simulink model "PassengerCar"  (R2019b)
settings: Solver=ode1  StartTime=0  StopTime=25  FixedStep=1.0000000000000000e-003  RelTol=1e-3
InitFcn:
  | sampleTime = str2double(get_param(bdroot, 'FixedStep'));
undefined symbols (not defined in the file or in its folder): AccPedalPos, BrakePedalPos, BrakeSwitch, DiscIntNeverNeededParam, DYNA4, EngSpd, IgnitionSwitch, InitialGear, InitialSpeed, IntendedEngTrq, LeftIndicator, MainBrakePress, MaxGear, MDL, MinGear, RefAcc, RefLane, RefLatPos, RefPath, RefPathCurv, RefSpd, RefSpdPreview, RefSpdRetrospect, RightIndicator, SteeringWheelAng, SteeringWheelTrq, UserDefinedRefValue, vm_const
libraries: UtilitiesLibrary x31, simulink x18, WheelSystemModules x13, LongitudinalControllerModules x13, LateralControllerModules x7, AnimationBusselectorModules x5, EnvironmentModules x5, BasicEngineControlModules x5, MiscellaneousControlModules x5, Animation3Modules x4, AuxiliariesModules x4, TireModules x4
(part 19 of 39)

== system PassengerCar/Vehicle/Engine/EngineControlUnit/EngineControlUnitOutput ==
  StarterSwitch[0;1]___UNIQUE_1 : Inport  Description=|  PortDimensions=[1]
      | <name>StarterSwitch[0;1]</name>
      | <comment>Engine starter switch</comment>
  EngRunPermission[0;1]___UNIQUE_1 : Inport  Description=|  Port=2  PortDimensions=[1]
      | <name>EngRunPermission[0;1]</name>
      | <comment>Switch indicating a engine stop due to start stop function or ignition off</comment>
  EngLoadSignal[0_1]___UNIQUE_1 : Inport  Description=|  Port=3  PortDimensions=[1]
      | <name>EngLoadSignal[0_1]</name>
      | <comment>Engine load signal</comment>
  EngIdleSpd[rad/s]___UNIQUE_1 : Inport  Description=|  Port=4  PortDimensions=[1]
      | <name>EngIdleSpd[rad/s]</name>
      | <comment>Engine idle speed</comment>
  EngFuelCutoff[0;1]___UNIQUE_1 : Inport  Description=|  Port=5  PortDimensions=[1]
      | <name>EngFuelCutoff[0;1]</name>
      | <comment>Logical signal which is true if fuel mass flow is stopped</comment>
  MaxEngSpd[rad/s]___UNIQUE_1 : Inport  Description=|  Port=6  PortDimensions=[1]
      | <name>MaxEngSpd[rad/s]</name>
      | <comment>Maximum allowed engine speed, threshold for fuel cut off</comment>
  UpperEngTrqSwitch[0;2]___UNIQUE_1 : Inport  Description=|  Port=7  PortDimensions=[1]
      | <name>UpperEngTrqSwitch[0;2]</name>
      | <comment>Switch indicating how the upper engine torque should be restricted (0: off, 1: slow, 2: fast)</comment>
  UpperEngTrqLimit[Nm]___UNIQUE_1 : Inport  Description=|  Port=8  PortDimensions=[1]
      | <name>UpperEngTrqLimit[Nm]</name>
      | <comment>Upper limit for the engine torque</comment>
  LowerEngTrqSwitch[0;2]___UNIQUE_1 : Inport  Description=|  Port=9  PortDimensions=[1]
      | <name>LowerEngTrqSwitch[0;2]</name>
      | <comment>Switch indicating how the lower engine torque should be restricted (0: off, 1: slow, 2: fast)</comment>
  LowerEngTrqLimit[Nm]___UNIQUE_1 : Inport  Description=|  Port=10  PortDimensions=[1]
      | <name>LowerEngTrqLimit[Nm]</name>
      | <comment>Lower limit for the engine torque</comment>
  __TDD__EngineControlUnit.EngFuelCutoff[0;1] : Demux  Outputs=[1]
  __TDD__EngineControlUnit.EngIdleSpd[rad/s] : Demux  Outputs=[1]
  __TDD__EngineControlUnit.EngLoadSignal[0_1] : Demux  Outputs=[1]
  __TDD__EngineControlUnit.EngRunPermission[0;1] : Demux  Outputs=[1]
  __TDD__EngineControlUnit.LowerEngTrqLimit[Nm] : Demux  Outputs=[1]
  __TDD__EngineControlUnit.LowerEngTrqSwitch[0;2] : Demux  Outputs=[1]
  __TDD__EngineControlUnit.MaxEngSpd[rad/s] : Demux  Outputs=[1]
  __TDD__EngineControlUnit.StarterSwitch[0;1] : Demux  Outputs=[1]
  __TDD__EngineControlUnit.UpperEngTrqLimit[Nm] : Demux  Outputs=[1]
  __TDD__EngineControlUnit.UpperEngTrqSwitch[0;2] : Demux  Outputs=[1]
  __TDO__EngineControlUnit : BusCreator  Inputs=10
  EngineControlUnit___UNIQUE_1 : Outport  Description=|  PortDimensions=[10]  VectorParamsAs1DForOutWhenUnconnected=off
      | <name>StarterSwitch[0;1]</name>
      | <comment>Engine starter switch</comment>
  wires:
  __TDO__EngineControlUnit/1 -> EngineControlUnit___UNIQUE_1/1  "EngineControlUnit"
  __TDD__EngineControlUnit.LowerEngTrqLimit[Nm]/1 -> __TDO__EngineControlUnit/10  "LowerEngTrqLimit[Nm]"
  LowerEngTrqLimit[Nm]___UNIQUE_1/1 -> __TDD__EngineControlUnit.LowerEngTrqLimit[Nm]/1
  __TDD__EngineControlUnit.LowerEngTrqSwitch[0;2]/1 -> __TDO__EngineControlUnit/9  "LowerEngTrqSwitch[0;2]"
  LowerEngTrqSwitch[0;2]___UNIQUE_1/1 -> __TDD__EngineControlUnit.LowerEngTrqSwitch[0;2]/1
  __TDD__EngineControlUnit.UpperEngTrqLimit[Nm]/1 -> __TDO__EngineControlUnit/8  "UpperEngTrqLimit[Nm]"
  UpperEngTrqLimit[Nm]___UNIQUE_1/1 -> __TDD__EngineControlUnit.UpperEngTrqLimit[Nm]/1
  __TDD__EngineControlUnit.UpperEngTrqSwitch[0;2]/1 -> __TDO__EngineControlUnit/7  "UpperEngTrqSwitch[0;2]"
  UpperEngTrqSwitch[0;2]___UNIQUE_1/1 -> __TDD__EngineControlUnit.UpperEngTrqSwitch[0;2]/1
  __TDD__EngineControlUnit.MaxEngSpd[rad/s]/1 -> __TDO__EngineControlUnit/6  "MaxEngSpd[rad/s]"
  MaxEngSpd[rad/s]___UNIQUE_1/1 -> __TDD__EngineControlUnit.MaxEngSpd[rad/s]/1
  __TDD__EngineControlUnit.EngFuelCutoff[0;1]/1 -> __TDO__EngineControlUnit/5  "EngFuelCutoff[0;1]"
  EngFuelCutoff[0;1]___UNIQUE_1/1 -> __TDD__EngineControlUnit.EngFuelCutoff[0;1]/1
  __TDD__EngineControlUnit.EngIdleSpd[rad/s]/1 -> __TDO__EngineControlUnit/4  "EngIdleSpd[rad/s]"
  EngIdleSpd[rad/s]___UNIQUE_1/1 -> __TDD__EngineControlUnit.EngIdleSpd[rad/s]/1
  __TDD__EngineControlUnit.EngLoadSignal[0_1]/1 -> __TDO__EngineControlUnit/3  "EngLoadSignal[0_1]"
  EngLoadSignal[0_1]___UNIQUE_1/1 -> __TDD__EngineControlUnit.EngLoadSignal[0_1]/1
  __TDD__EngineControlUnit.EngRunPermission[0;1]/1 -> __TDO__EngineControlUnit/2  "EngRunPermission[0;1]"
  EngRunPermission[0;1]___UNIQUE_1/1 -> __TDD__EngineControlUnit.EngRunPermission[0;1]/1
  __TDD__EngineControlUnit.StarterSwitch[0;1]/1 -> __TDO__EngineControlUnit/1  "StarterSwitch[0;1]"
  StarterSwitch[0;1]___UNIQUE_1/1 -> __TDD__EngineControlUnit.StarterSwitch[0;1]/1

== system PassengerCar/Vehicle/Engine/EngineControlUnit/InputFromCTRL ==
  fromCTRL : Inport
  TDBusSelector : BusSelector  OutputSignals=CTRL.LongitudinalControl.IgnitionSwitch[0;3],CTRL.LongitudinalControl.EngRunPermission[0;1],CTRL.LongitudinalControl.AccPedalPos[0_1],CTRL.LongitudinalControl.IntendedEngTrq[Nm],CTRL.LongitudinalControl.IntendedEngTrqActive[0;1],CTRL.LongitudinalControl.ClutchPos[0_1]
  __TDD__AccPedalPos[0_1] : Demux  Outputs=1
  __TDD__ClutchPos[0_1] : Demux  Outputs=[1]
  __TDD__EngRunPermission[0;1] : Demux  Outputs=[1]
  __TDD__IgnitionSwitch[0;3] : Demux  Outputs=[1]
  __TDD__IntendedEngTrqActive[0;1] : Demux  Outputs=[1]
  __TDD__IntendedEngTrq[Nm] : Demux  Outputs=[1]
  IgnitionSwitch[0;3]___UNIQUE_1 : Outport  Description=|  PortDimensions=[1]  VectorParamsAs1DForOutWhenUnconnected=off
      | <name>CTRL.LongitudinalControl.IgnitionSwitch[0;3]</name>
      | <comment>Ignition signal with four signal states: 0 - ignition off + consumer off + starter off, 1 - ignition off + consumer on + starter off, 2 - ignition on + consumer on + starter off, 3 - ignition on + consumer on  + starter on</comment>
  EngRunPermission[0;1]___UNIQUE_1 : Outport  Description=|  Port=2  PortDimensions=[1]  VectorParamsAs1DForOutWhenUnconnected=off
      | <name>CTRL.LongitudinalControl.EngRunPermission[0;1]</name>
      | <comment></comment>
  AccPedalPos[0_1]___UNIQUE_1 : Outport  Description=|  Port=3  VectorParamsAs1DForOutWhenUnconnected=off
      | <name>CTRL.LongitudinalControl.AccPedalPos[0_1]</name>
      | <comment></comment>
  IntendedEngTrq[Nm]___UNIQUE_1 : Outport  Description=|  Port=4  PortDimensions=[1]  VectorParamsAs1DForOutWhenUnconnected=off
      | <name>CTRL.LongitudinalControl.IntendedEngTrq[Nm]</name>
      | <comment></comment>
  IntendedEngTrqActive[0;1]___UNIQUE_1 : Outport  Description=|  Port=5  PortDimensions=[1]  VectorParamsAs1DForOutWhenUnconnected=off
      | <name>CTRL.LongitudinalControl.IntendedEngTrqActive[0;1]</name>
      | <comment></comment>
  ClutchPos[0_1]___UNIQUE_1 : Outport  Description=|  Port=6  PortDimensions=[1]  VectorParamsAs1DForOutWhenUnconnected=off
      | <name>CTRL.LongitudinalControl.ClutchPos[0_1]</name>
      | <comment>Clutch position</comment>
  wires:
  __TDD__ClutchPos[0_1]/1 -> ClutchPos[0_1]___UNIQUE_1/1  "ClutchPos[0_1]"
  __TDD__IntendedEngTrqActive[0;1]/1 -> IntendedEngTrqActive[0;1]___UNIQUE_1/1  "IntendedEngTrqActive[0;1]"
  __TDD__IntendedEngTrq[Nm]/1 -> IntendedEngTrq[Nm]___UNIQUE_1/1  "IntendedEngTrq[Nm]"
  __TDD__AccPedalPos[0_1]/1 -> AccPedalPos[0_1]___UNIQUE_1/1  "AccPedalPos[0_1]"
  __TDD__EngRunPermission[0;1]/1 -> EngRunPermission[0;1]___UNIQUE_1/1  "EngRunPermission[0;1]"
  __TDD__IgnitionSwitch[0;3]/1 -> IgnitionSwitch[0;3]___UNIQUE_1/1  "IgnitionSwitch[0;3]"
  TDBusSelector/6 -> __TDD__ClutchPos[0_1]/1  "<ClutchPos[0_1]>"
  TDBusSelector/5 -> __TDD__IntendedEngTrqActive[0;1]/1  "<IntendedEngTrqActive[0;1]>"
  TDBusSelector/4 -> __TDD__IntendedEngTrq[Nm]/1  "<IntendedEngTrq[Nm]>"
  TDBusSelector/3 -> __TDD__AccPedalPos[0_1]/1  "<AccPedalPos[0_1]>"
  TDBusSelector/2 -> __TDD__EngRunPermission[0;1]/1  "<EngRunPermission[0;1]>"
  TDBusSelector/1 -> __TDD__IgnitionSwitch[0;3]/1  "<IgnitionSwitch[0;3]>"
  fromCTRL/1 -> TDBusSelector/1

== system PassengerCar/Vehicle/Engine/EngineControlUnit/InputFromCTRL1 ==
  fromCTRL : Inport
  TDBusSelector : BusSelector  OutputSignals=CTRL.LongitudinalControl.ASRRequestSwitch[0;2],CTRL.LongitudinalControl.ASRTrq[Nm],CTRL.LongitudinalControl.MSRRequestSwitch[0;2],CTRL.LongitudinalControl.MSRTrq[Nm]
  __TDD__ASRRequestSwitch[0;2] : Demux  Outputs=1
  __TDD__ASRTrq[Nm] : Demux  Outputs=1
  __TDD__MSRRequestSwitch[0;2] : Demux  Outputs=1
  __TDD__MSRTrq[Nm] : Demux  Outputs=1
  ASRRequestSwitch[0;2]___UNIQUE_1 : Outport  Description=|  VectorParamsAs1DForOutWhenUnconnected=off
      | <name>CTRL.LongitudinalControl.ASRRequestSwitch[0;2]</name>
      | <comment></comment>
  ASRTrq[Nm]___UNIQUE_1 : Outport  Description=|  Port=2  VectorParamsAs1DForOutWhenUnconnected=off
      | <name>CTRL.LongitudinalControl.ASRTrq[Nm]</name>
      | <comment></comment>
  MSRRequestSwitch[0;2]___UNIQUE_1 : Outport  Description=|  Port=3  VectorParamsAs1DForOutWhenUnconnected=off
      | <name>CTRL.LongitudinalControl.MSRRequestSwitch[0;2]</name>
      | <comment></comment>
  MSRTrq[Nm]___UNIQUE_1 : Outport  Description=|  Port=4  VectorParamsAs1DForOutWhenUnconnected=off
      | <name>CTRL.LongitudinalControl.MSRTrq[Nm]</name>
      | <comment></comment>
  wires:
  __TDD__MSRTrq[Nm]/1 -> MSRTrq[Nm]___UNIQUE_1/1  "MSRTrq[Nm]"
  __TDD__MSRRequestSwitch[0;2]/1 -> MSRRequestSwitch[0;2]___UNIQUE_1/1  "MSRRequestSwitch[0;2]"
  __TDD__ASRTrq[Nm]/1 -> ASRTrq[Nm]___UNIQUE_1/1  "ASRTrq[Nm]"
  __TDD__ASRRequestSwitch[0;2]/1 -> ASRRequestSwitch[0;2]___UNIQUE_1/1  "ASRRequestSwitch[0;2]"
  TDBusSelector/4 -> __TDD__MSRTrq[Nm]/1  "<MSRTrq[Nm]>"
  TDBusSelector/3 -> __TDD__MSRRequestSwitch[0;2]/1  "<MSRRequestSwitch[0;2]>"
  TDBusSelector/2 -> __TDD__ASRTrq[Nm]/1  "<ASRTrq[Nm]>"
  TDBusSelector/1 -> __TDD__ASRRequestSwitch[0;2]/1  "<ASRRequestSwitch[0;2]>"
  fromCTRL/1 -> TDBusSelector/1

== system PassengerCar/Vehicle/Engine/EngineControlUnit/InputFromChassis ==
  fromChassis : Inport
  TDBusSelector : BusSelector  OutputSignals=VehicleBody.AbsVel[m/s]
  __TDD__AbsVel[m/s] : Demux  Outputs=1
  AbsVel[m/s]___UNIQUE_1 : Outport  Description=|  VectorParamsAs1DForOutWhenUnconnected=off
      | <name>VehicleBody.AbsVel[m/s]</name>
      | <comment></comment>
  wires:
  __TDD__AbsVel[m/s]/1 -> AbsVel[m/s]___UNIQUE_1/1  "AbsVel[m/s]"
  TDBusSelector/1 -> __TDD__AbsVel[m/s]/1  "<AbsVel[m/s]>"
  fromChassis/1 -> TDBusSelector/1

== system PassengerCar/Vehicle/Engine/EngineControlUnit/InputFromDrivetrain ==
  fromDrivetrain : Inport
  TDBusSelector : BusSelector  OutputSignals=DrivetrainPhysics.Transmission.Gear[-4;20],DrivetrainPhysics.EngSpd[rad/s]
  __TDD__EngSpd[rad/s] : Demux  Outputs=1
  __TDD__Gear[-4;20] : Demux  Outputs=1
  Gear[-4;20] : Outport  Description=|  VectorParamsAs1DForOutWhenUnconnected=off
      | <name>DrivetrainPhysics.Transmission.Gear[-4;20]</name>
      | <comment></comment>
  EngSpd[rad/s] : Outport  Description=|  Port=2  VectorParamsAs1DForOutWhenUnconnected=off
      | <name>DrivetrainPhysics.EngSpd[rad/s]</name>
      | <comment></comment>
  wires:
  __TDD__EngSpd[rad/s]/1 -> EngSpd[rad/s]/1  "EngSpd[rad/s]"
  __TDD__Gear[-4;20]/1 -> Gear[-4;20]/1  "Gear[-4;20]"
  TDBusSelector/2 -> __TDD__EngSpd[rad/s]/1  "<EngSpd[rad/s]>"
  TDBusSelector/1 -> __TDD__Gear[-4;20]/1  "<Gear[-4;20]>"
  fromDrivetrain/1 -> TDBusSelector/1

== system PassengerCar/Vehicle/Engine/EngineControlUnit/InputFromEnginePhysics ==
  fromEnginePhysics : Inport
  TDBusSelector : BusSelector  OutputSignals=Mechanics.EngTrq[Nm],Mechanics.UnrestrictedEngTrq[Nm],Mechanics.MeanEngFrictionTrq[Nm],Mechanics.MeanEngMaxTrq[Nm]
  __TDD__EngTrq[Nm] : Demux  Outputs=[1]
  __TDD__MeanEngFrictionTrq[Nm] : Demux  Outputs=1
  __TDD__MeanEngMaxTrq[Nm] : Demux  Outputs=1
  __TDD__UnrestrictedEngTrq[Nm] : Demux  Outputs=[1]
  EngTrq[Nm]___UNIQUE_1 : Outport  Description=|  PortDimensions=[1]  VectorParamsAs1DForOutWhenUnconnected=off
      | <name>Mechanics.EngTrq[Nm]</name>
      | <comment>Engine torque</comment>
  UnrestrictedEngTrq[Nm]___UNIQUE_1 : Outport  Description=|  Port=2  PortDimensions=[1]  VectorParamsAs1DForOutWhenUnconnected=off
      | <name>Mechanics.UnrestrictedEngTrq[Nm]</name>
      | <comment>Unrestricted engine torque</comment>
  MeanEngFrictionTrq[Nm]___UNIQUE_1 : Outport  Description=|  Port=3  VectorParamsAs1DForOutWhenUnconnected=off
      | <name>Mechanics.MeanEngFrictionTrq[Nm]</name>
      | <comment></comment>
  MeanEngMaxTrq[Nm]___UNIQUE_1 : Outport  Description=|  Port=4  VectorParamsAs1DForOutWhenUnconnected=off
      | <name>Mechanics.MeanEngMaxTrq[Nm]</name>
      | <comment></comment>
  wires:
  __TDD__MeanEngMaxTrq[Nm]/1 -> MeanEngMaxTrq[Nm]___UNIQUE_1/1  "MeanEngMaxTrq[Nm]"
  __TDD__MeanEngFrictionTrq[Nm]/1 -> MeanEngFrictionTrq[Nm]___UNIQUE_1/1  "MeanEngFrictionTrq[Nm]"
  __TDD__UnrestrictedEngTrq[Nm]/1 -> UnrestrictedEngTrq[Nm]___UNIQUE_1/1  "UnrestrictedEngTrq[Nm]"
  __TDD__EngTrq[Nm]/1 -> EngTrq[Nm]___UNIQUE_1/1  "EngTrq[Nm]"
  TDBusSelector/4 -> __TDD__MeanEngMaxTrq[Nm]/1  "<MeanEngMaxTrq[Nm]>"
  TDBusSelector/3 -> __TDD__MeanEngFrictionTrq[Nm]/1  "<MeanEngFrictionTrq[Nm]>"
  TDBusSelector/2 -> __TDD__UnrestrictedEngTrq[Nm]/1  "<UnrestrictedEngTrq[Nm]>"
  TDBusSelector/1 -> __TDD__EngTrq[Nm]/1  "<EngTrq[Nm]>"
  fromEnginePhysics/1 -> TDBusSelector/1

== system PassengerCar/Vehicle/Engine/EnginePhysics/DynaComponentInfo ==

== system PassengerCar/Vehicle/Engine/EnginePhysics/EnginePhysicsOutput ==
  Mechanics___UNIQUE_1 : Inport  Description=|
      | <name>Mechanics</name>
      | <comment></comment>
  ValidityStatus___UNIQUE_1 : Inport  Description=|  Port=2
      | <name>ValidityStatus</name>
      | <comment></comment>
  FuelSystem___UNIQUE_1 : Inport  Description=|  Port=3
      | <name>FuelSystem</name>
      | <comment></comment>
  __TDO__EnginePhysics : BusCreator  Inputs=3
  EnginePhysics___UNIQUE_1 : Outport  Description=|  VectorParamsAs1DForOutWhenUnconnected=off
      | <name>Mechanics</name>
      | <comment></comment>
  wires:
  __TDO__EnginePhysics/1 -> EnginePhysics___UNIQUE_1/1  "EnginePhysics"
  FuelSystem___UNIQUE_1/1 -> __TDO__EnginePhysics/3  "FuelSystem"
  ValidityStatus___UNIQUE_1/1 -> __TDO__EnginePhysics/2  "ValidityStatus"
  Mechanics___UNIQUE_1/1 -> __TDO__EnginePhysics/1  "Mechanics"

== system PassengerCar/Vehicle/Engine/EnginePhysics/FuelSystemOutput ==
  FuelMassFlow[kg/s]___UNIQUE_1 : Inport  Description=|  PortDimensions=[1]
      | <name>FuelMassFlow[kg/s]</name>
      | <comment></comment>
  FuelMass[kg]___UNIQUE_1 : Inport  Description=|  Port=2  PortDimensions=[1]
      | <name>FuelMass[kg]</name>
      | <comment></comment>
  CurrFuelConsumEu[l/100km]___UNIQUE_1 : Inport  Description=|  Port=3  PortDimensions=[1]
      | <name>CurrFuelConsumEu[l/100km]</name>
      | <comment></comment>
  CurrFuelConsumUs[mpg]___UNIQUE_1 : Inport  Description=|  Port=4  PortDimensions=[1]
      | <name>CurrFuelConsumUs[mpg]</name>
      | <comment></comment>
  AvgFuelConsumEu[l/100km]___UNIQUE_1 : Inport  Description=|  Port=5  PortDimensions=[1]
      | <name>AvgFuelConsumEu[l/100km]</name>
      | <comment></comment>
  AvgFuelConsumUs[mpg]___UNIQUE_1 : Inport  Description=|  Port=6  PortDimensions=[1]
      | <name>AvgFuelConsumUs[mpg]</name>
      | <comment></comment>
  Efficiency[-]___UNIQUE_1 : Inport  Description=|  Port=7  PortDimensions=[1]
      | <name>Efficiency[-]</name>
      | <comment></comment>
  FuelDensity[kg/m**3]___UNIQUE_1 : Inport  Description=|  Port=8  PortDimensions=[1]
      | <name>FuelDensity[kg/m**3]</name>
      | <comment></comment>
  __TDD__FuelSystem.AvgFuelConsumEu[l/100km] : Demux  Outputs=[1]
  __TDD__FuelSystem.AvgFuelConsumUs[mpg] : Demux  Outputs=[1]
  __TDD__FuelSystem.CurrFuelConsumEu[l/100km] : Demux  Outputs=[1]
  __TDD__FuelSystem.CurrFuelConsumUs[mpg] : Demux  Outputs=[1]
  __TDD__FuelSystem.Efficiency[-] : Demux  Outputs=[1]
  __TDD__FuelSystem.FuelDensity[kg/m**3] : Demux  Outputs=[1]
  __TDD__FuelSystem.FuelMassFlow[kg/s] : Demux  Outputs=[1]
  __TDD__FuelSystem.FuelMass[kg] : Demux  Outputs=[1]
  __TDO__FuelSystem : BusCreator  Inputs=8
  FuelSystem___UNIQUE_1 : Outport  Description=|  PortDimensions=[8]  VectorParamsAs1DForOutWhenUnconnected=off
      | <name>FuelMassFlow[kg/s]</name>
      | <comment></comment>
  wires:
  __TDO__FuelSystem/1 -> FuelSystem___UNIQUE_1/1  "FuelSystem"
  __TDD__FuelSystem.FuelDensity[kg/m**3]/1 -> __TDO__FuelSystem/8  "FuelDensity[kg/m**3]"
  FuelDensity[kg/m**3]___UNIQUE_1/1 -> __TDD__FuelSystem.FuelDensity[kg/m**3]/1
  __TDD__FuelSystem.Efficiency[-]/1 -> __TDO__FuelSystem/7  "Efficiency[-]"
  Efficiency[-]___UNIQUE_1/1 -> __TDD__FuelSystem.Efficiency[-]/1
  __TDD__FuelSystem.AvgFuelConsumUs[mpg]/1 -> __TDO__FuelSystem/6  "AvgFuelConsumUs[mpg]"
  AvgFuelConsumUs[mpg]___UNIQUE_1/1 -> __TDD__FuelSystem.AvgFuelConsumUs[mpg]/1
  __TDD__FuelSystem.AvgFuelConsumEu[l/100km]/1 -> __TDO__FuelSystem/5  "AvgFuelConsumEu[l/100km]"
  AvgFuelConsumEu[l/100km]___UNIQUE_1/1 -> __TDD__FuelSystem.AvgFuelConsumEu[l/100km]/1
  __TDD__FuelSystem.CurrFuelConsumUs[mpg]/1 -> __TDO__FuelSystem/4  "CurrFuelConsumUs[mpg]"
  CurrFuelConsumUs[mpg]___UNIQUE_1/1 -> __TDD__FuelSystem.CurrFuelConsumUs[mpg]/1
  __TDD__FuelSystem.CurrFuelConsumEu[l/100km]/1 -> __TDO__FuelSystem/3  "CurrFuelConsumEu[l/100km]"
  CurrFuelConsumEu[l/100km]___UNIQUE_1/1 -> __TDD__FuelSystem.CurrFuelConsumEu[l/100km]/1
  __TDD__FuelSystem.FuelMass[kg]/1 -> __TDO__FuelSystem/2  "FuelMass[kg]"
  FuelMass[kg]___UNIQUE_1/1 -> __TDD__FuelSystem.FuelMass[kg]/1
  __TDD__FuelSystem.FuelMassFlow[kg/s]/1 -> __TDO__FuelSystem/1  "FuelMassFlow[kg/s]"
  FuelMassFlow[kg/s]___UNIQUE_1/1 -> __TDD__FuelSystem.FuelMassFlow[kg/s]/1

== system PassengerCar/Vehicle/Engine/EnginePhysics/InputFromChassis ==
  fromChassis : Inport
  TDBusSelector : BusSelector  OutputSignals=VehicleBody.AbsVel[m/s]
  __TDD__AbsVel[m/s] : Demux  Outputs=1
  AbsVel[m/s]___UNIQUE_1 : Outport  Description=|  VectorParamsAs1DForOutWhenUnconnected=off
      | <name>VehicleBody.AbsVel[m/s]</name>
      | <comment></comment>
  wires:
  __TDD__AbsVel[m/s]/1 -> AbsVel[m/s]___UNIQUE_1/1  "AbsVel[m/s]"
  TDBusSelector/1 -> __TDD__AbsVel[m/s]/1  "<AbsVel[m/s]>"
  fromChassis/1 -> TDBusSelector/1

== system PassengerCar/Vehicle/Engine/EnginePhysics/InputFromDrivetrain ==
  fromDrivetrain : Inport
  TDBusSelector : BusSelector  OutputSignals=DrivetrainPhysics.EngSpd[rad/s]
  __TDD__EngSpd[rad/s] : Demux  Outputs=1
  EngSpd[rad/s] : Outport  Description=|  VectorParamsAs1DForOutWhenUnconnected=off
      | <name>DrivetrainPhysics.EngSpd[rad/s]</name>
      | <comment></comment>
  wires:
  __TDD__EngSpd[rad/s]/1 -> EngSpd[rad/s]/1  "EngSpd[rad/s]"
  TDBusSelector/1 -> __TDD__EngSpd[rad/s]/1  "<EngSpd[rad/s]>"
  fromDrivetrain/1 -> TDBusSelector/1

== system PassengerCar/Vehicle/Engine/EnginePhysics/InputFromEngineControlUnit ==
  fromEngineControlUnit : Inport
  TDBusSelector : BusSelector  OutputSignals=EngLoadSignal[0_1],EngFuelCutoff[0;1],UpperEngTrqSwitch[0;2],UpperEngTrqLimit[Nm],LowerEngTrqSwitch[0;2],LowerEngTrqLimit[Nm]
  __TDD__EngFuelCutoff[0;1] : Demux  Outputs=1
  __TDD__EngLoadSignal[0_1] : Demux  Outputs=1
  __TDD__LowerEngTrqLimit[Nm] : Demux  Outputs=1
  __TDD__LowerEngTrqSwitch[0;2] : Demux  Outputs=1
  __TDD__UpperEngTrqLimit[Nm] : Demux  Outputs=1
  __TDD__UpperEngTrqSwitch[0;2] : Demux  Outputs=1
  EngLoadSignal[0_1]___UNIQUE_1 : Outport  Description=|  VectorParamsAs1DForOutWhenUnconnected=off
      | <name>EngLoadSignal[0_1]</name>
      | <comment></comment>
  EngFuelCutoff[0;1]___UNIQUE_1 : Outport  Description=|  Port=2  VectorParamsAs1DForOutWhenUnconnected=off
      | <name>EngFuelCutoff[0;1]</name>
      | <comment></comment>
  UpperEngTrqSwitch[0;2]___UNIQUE_1 : Outport  Description=|  Port=3  VectorParamsAs1DForOutWhenUnconnected=off
      | <name>UpperEngTrqSwitch[0;2]</name>
      | <comment></comment>
  UpperEngTrqLimit[Nm]___UNIQUE_1 : Outport  Description=|  Port=4  VectorParamsAs1DForOutWhenUnconnected=off
      | <name>UpperEngTrqLimit[Nm]</name>
      | <comment></comment>
  LowerEngTrqSwitch[0;2]___UNIQUE_1 : Outport  Description=|  Port=5  VectorParamsAs1DForOutWhenUnconnected=off
      | <name>LowerEngTrqSwitch[0;2]</name>
      | <comment></comment>
  LowerEngTrqLimit[Nm]___UNIQUE_1 : Outport  Description=|  Port=6  VectorParamsAs1DForOutWhenUnconnected=off
      | <name>LowerEngTrqLimit[Nm]</name>
      | <comment></comment>
  wires:
  __TDD__LowerEngTrqLimit[Nm]/1 -> LowerEngTrqLimit[Nm]___UNIQUE_1/1  "LowerEngTrqLimit[Nm]"
  __TDD__LowerEngTrqSwitch[0;2]/1 -> LowerEngTrqSwitch[0;2]___UNIQUE_1/1  "LowerEngTrqSwitch[0;2]"
  __TDD__UpperEngTrqLimit[Nm]/1 -> UpperEngTrqLimit[Nm]___UNIQUE_1/1  "UpperEngTrqLimit[Nm]"
  __TDD__UpperEngTrqSwitch[0;2]/1 -> UpperEngTrqSwitch[0;2]___UNIQUE_1/1  "UpperEngTrqSwitch[0;2]"
  __TDD__EngFuelCutoff[0;1]/1 -> EngFuelCutoff[0;1]___UNIQUE_1/1  "EngFuelCutoff[0;1]"
  __TDD__EngLoadSignal[0_1]/1 -> EngLoadSignal[0_1]___UNIQUE_1/1  "EngLoadSignal[0_1]"
  TDBusSelector/6 -> __TDD__LowerEngTrqLimit[Nm]/1  "<LowerEngTrqLimit[Nm]>"
  TDBusSelector/5 -> __TDD__LowerEngTrqSwitch[0;2]/1  "<LowerEngTrqSwitch[0;2]>"
  TDBusSelector/4 -> __TDD__UpperEngTrqLimit[Nm]/1  "<UpperEngTrqLimit[Nm]>"
  TDBusSelector/3 -> __TDD__UpperEngTrqSwitch[0;2]/1  "<UpperEngTrqSwitch[0;2]>"
  TDBusSelector/2 -> __TDD__EngFuelCutoff[0;1]/1  "<EngFuelCutoff[0;1]>"
  TDBusSelector/1 -> __TDD__EngLoadSignal[0_1]/1  "<EngLoadSignal[0_1]>"
  fromEngineControlUnit/1 -> TDBusSelector/1

== system PassengerCar/Vehicle/Engine/EnginePhysics/MechanicsOutput ==
  EngTrq[Nm]___UNIQUE_1 : Inport  Description=|  PortDimensions=[1]
      | <name>EngTrq[Nm]</name>
      | <comment></comment>
  MeanEngTrq[Nm]___UNIQUE_1 : Inport  Description=|  Port=2  PortDimensions=[1]
      | <name>MeanEngTrq[Nm]</name>
      | <comment></comment>
  IndicatedTrq[Nm]___UNIQUE_1 : Inport  Description=|  Port=3  PortDimensions=[1]
      | <name>IndicatedTrq[Nm]</name>
      | <comment></comment>
  MeanIndicatedTrq[Nm]___UNIQUE_1 : Inport  Description=|  Port=4  PortDimensions=[1]
      | <name>MeanIndicatedTrq[Nm]</name>
      | <comment></comment>
  MeanEngFrictionTrq[Nm]___UNIQUE_1 : Inport  Description=|  Port=5  PortDimensions=[1]
      | <name>MeanEngFrictionTrq[Nm]</name>
      | <comment></comment>
  MeanEngDragTrq[Nm]___UNIQUE_1 : Inport  Description=|  Port=6  PortDimensions=[1]
      | <name>MeanEngDragTrq[Nm]</name>
      | <comment></comment>
  UnrestrictedEngTrq[Nm]___UNIQUE_1 : Inport  Description=|  Port=7  PortDimensions=[1]
      | <name>UnrestrictedEngTrq[Nm]</name>
      | <comment></comment>
  EngPow[W]___UNIQUE_1 : Inport  Description=|  Port=8  PortDimensions=[1]
      | <name>EngPow[W]</name>
      | <comment></comment>
  EngInrt[kg*m**2]___UNIQUE_1 : Inport  Description=|  Port=9  PortDimensions=[1]
      | <name>EngInrt[kg*m**2]</name>
      | <comment></comment>
  MeanEngMaxTrq[Nm]___UNIQUE_1 : Inport  Description=|  Port=10  PortDimensions=[1]
      | <name>MeanEngMaxTrq[Nm]</name>
      | <comment></comment>
  ThirtyPercentAccPedalEngTrq[Nm]___UNIQUE_1 : Inport  Description=|  Port=11  PortDimensions=[1]
      | <name>ThirtyPercentAccPedalEngTrq[Nm]</name>
      | <comment></comment>
  __SRC__Mechanics.CrankAng[rad] : Constant  Value=0.0  OutDataTypeStr=Inherit: Inherit via back propagation
  __SRC__Mechanics.DerivativeOfEngTrq_wrt_CrankAng[Nm/rad] : Constant  Value=0.0  OutDataTypeStr=Inherit: Inherit via back propagation
  __SRC__Mechanics.DerivativeOfEngTrq_wrt_EngSpd[Nm/(rad/s)] : Constant  Value=0.0  OutDataTypeStr=Inherit: Inherit via back propagation
  __TDD__Mechanics.EngInrt[kg*m**2] : Demux  Outputs=[1]
  __TDD__Mechanics.EngPow[W] : Demux  Outputs=[1]
  __TDD__Mechanics.EngTrq[Nm] : Demux  Outputs=[1]
  __TDD__Mechanics.IndicatedTrq[Nm] : Demux  Outputs=[1]
  __TDD__Mechanics.MeanEngDragTrq[Nm] : Demux  Outputs=[1]
  __TDD__Mechanics.MeanEngFrictionTrq[Nm] : Demux  Outputs=[1]
  __TDD__Mechanics.MeanEngMaxTrq[Nm] : Demux  Outputs=[1]
  __TDD__Mechanics.MeanEngTrq[Nm] : Demux  Outputs=[1]
  __TDD__Mechanics.MeanIndicatedTrq[Nm] : Demux  Outputs=[1]
  __TDD__Mechanics.ThirtyPercentAccPedalEngTrq[Nm] : Demux  Outputs=[1]
  __TDD__Mechanics.UnrestrictedEngTrq[Nm] : Demux  Outputs=[1]
  __TDO__Mechanics : BusCreator  Inputs=14
  Mechanics___UNIQUE_1 : Outport  Description=|  PortDimensions=[14]  VectorParamsAs1DForOutWhenUnconnected=off
      | <name>EngTrq[Nm]</name>
      | <comment></comment>
  wires:
  __TDO__Mechanics/1 -> Mechanics___UNIQUE_1/1  "Mechanics"
  __SRC__Mechanics.DerivativeOfEngTrq_wrt_EngSpd[Nm/(rad/s)]/1 -> __TDO__Mechanics/14  "DerivativeOfEngTrq_wrt_EngSpd[Nm/(rad/s)]"
  __SRC__Mechanics.DerivativeOfEngTrq_wrt_CrankAng[Nm/rad]/1 -> __TDO__Mechanics/13  "DerivativeOfEngTrq_wrt_CrankAng[Nm/rad]"
  __SRC__Mechanics.CrankAng[rad]/1 -> __TDO__Mechanics/12  "CrankAng[rad]"
  __TDD__Mechanics.ThirtyPercentAccPedalEngTrq[Nm]/1 -> __TDO__Mechanics/11  "ThirtyPercentAccPedalEngTrq[Nm]"
  ThirtyPercentAccPedalEngTrq[Nm]___UNIQUE_1/1 -> __TDD__Mechanics.ThirtyPercentAccPedalEngTrq[Nm]/1
  __TDD__Mechanics.MeanEngMaxTrq[Nm]/1 -> __TDO__Mechanics/10  "MeanEngMaxTrq[Nm]"
  MeanEngMaxTrq[Nm]___UNIQUE_1/1 -> __TDD__Mechanics.MeanEngMaxTrq[Nm]/1
  __TDD__Mechanics.EngInrt[kg*m**2]/1 -> __TDO__Mechanics/9  "EngInrt[kg*m**2]"
  EngInrt[kg*m**2]___UNIQUE_1/1 -> __TDD__Mechanics.EngInrt[kg*m**2]/1
  __TDD__Mechanics.EngPow[W]/1 -> __TDO__Mechanics/8  "EngPow[W]"
  EngPow[W]___UNIQUE_1/1 -> __TDD__Mechanics.EngPow[W]/1
  __TDD__Mechanics.UnrestrictedEngTrq[Nm]/1 -> __TDO__Mechanics/7  "UnrestrictedEngTrq[Nm]"
  UnrestrictedEngTrq[Nm]___UNIQUE_1/1 -> __TDD__Mechanics.UnrestrictedEngTrq[Nm]/1
  __TDD__Mechanics.MeanEngDragTrq[Nm]/1 -> __TDO__Mechanics/6  "MeanEngDragTrq[Nm]"
  MeanEngDragTrq[Nm]___UNIQUE_1/1 -> __TDD__Mechanics.MeanEngDragTrq[Nm]/1
  __TDD__Mechanics.MeanEngFrictionTrq[Nm]/1 -> __TDO__Mechanics/5  "MeanEngFrictionTrq[Nm]"
  MeanEngFrictionTrq[Nm]___UNIQUE_1/1 -> __TDD__Mechanics.MeanEngFrictionTrq[Nm]/1
  __TDD__Mechanics.MeanIndicatedTrq[Nm]/1 -> __TDO__Mechanics/4  "MeanIndicatedTrq[Nm]"
  MeanIndicatedTrq[Nm]___UNIQUE_1/1 -> __TDD__Mechanics.MeanIndicatedTrq[Nm]/1
  __TDD__Mechanics.IndicatedTrq[Nm]/1 -> __TDO__Mechanics/3  "IndicatedTrq[Nm]"
  IndicatedTrq[Nm]___UNIQUE_1/1 -> __TDD__Mechanics.IndicatedTrq[Nm]/1
  __TDD__Mechanics.MeanEngTrq[Nm]/1 -> __TDO__Mechanics/2  "MeanEngTrq[Nm]"
  MeanEngTrq[Nm]___UNIQUE_1/1 -> __TDD__Mechanics.MeanEngTrq[Nm]/1
  __TDD__Mechanics.EngTrq[Nm]/1 -> __TDO__Mechanics/1  "EngTrq[Nm]"
  EngTrq[Nm]___UNIQUE_1/1 -> __TDD__Mechanics.EngTrq[Nm]/1

== system PassengerCar/Vehicle/Engine/EnginePhysics/ValidityStatus ==
  ValidRangeExceededFlags[-]___UNIQUE_1 : Inport  Description=|  PortDimensions=[1]
      | <name>ValidRangeExceededFlags[-]</name>
      | <comment></comment>
  __TDD__ValidityStatus.ValidRangeExceededFlags[-] : Demux  Outputs=[1]
  __TDO__ValidityStatus : BusCreator  Inputs=1
  ValidityStatus___UNIQUE_1 : Outport  Description=|  PortDimensions=[1]  VectorParamsAs1DForOutWhenUnconnected=off
      | <name>ValidRangeExceededFlags[-]</name>
      | <comment></comment>
  wires:
  __TDO__ValidityStatus/1 -> ValidityStatus___UNIQUE_1/1  "ValidityStatus"
  __TDD__ValidityStatus.ValidRangeExceededFlags[-]/1 -> __TDO__ValidityStatus/1  "ValidRangeExceededFlags[-]"
  ValidRangeExceededFlags[-]___UNIQUE_1/1 -> __TDD__ValidityStatus.ValidRangeExceededFlags[-]/1

== system PassengerCar/Vehicle/VehicleRoadInfo/AdditionalRoadElevationAndRoadSlopes/Convert2VehSys ==
  note: RoadSlope(VehSys) = LongRoadSlope(WorldSys)*cos(yaw) + LatRoadSlope(WorldSys)*sin(yaw)
  YawAng[rad] : Inport
  RoadSlopes(WorldSys) : Inport  Port=2
  Demux3 : Demux  Outputs=2
  Product : Product
  Product1 : Product
  Sum : Sum
  Trigonometric Function : Trigonometry
  Trigonometric Function1 : Trigonometry  Operator=cos
  RoadSlopes(VehSys) : Outport  VectorParamsAs1DForOutWhenUnconnected=off
  wires:
  Sum/1 -> RoadSlopes(VehSys)/1
  Product/1 -> Sum/2
  Product1/1 -> Sum/1
  Trigonometric Function1/1 -> Product1/1
  Demux3/2 -> Product/2  "LatRoadSlope"
  Trigonometric Function/1 -> Product/1
  YawAng[rad]/1 -> Trigonometric Function1/1, Trigonometric Function/1
  Demux3/1 -> Product1/2  "LongRoadSlope"
  RoadSlopes(WorldSys)/1 -> Demux3/1

== system PassengerCar/Vehicle/WheelSystem/FrontLeftWheelSystem/DynaSystemInfo ==

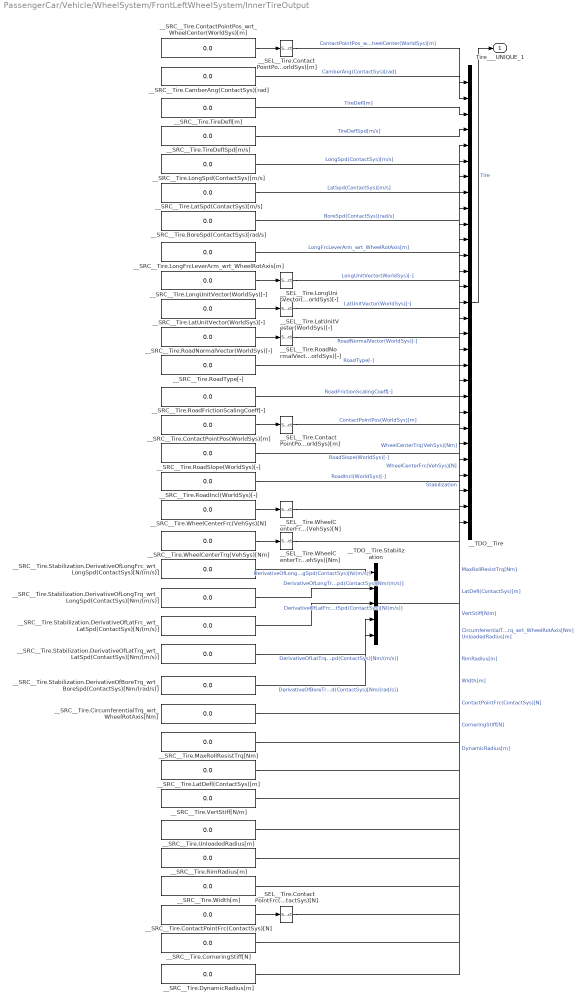
== system PassengerCar/Vehicle/WheelSystem/FrontLeftWheelSystem/InnerTireOutput ==
  __SEL__Tire.ContactPointFrc(ContactSys)[N] : Selector  InputPortWidth=1  IndexOptions=Index vector (dialog)  Indices=ones(3, 1)  OutputSizes=1
  __SEL__Tire.ContactPointPos(WorldSys)[m] : Selector  InputPortWidth=1  IndexOptions=Index vector (dialog)  Indices=ones(3, 1)  OutputSizes=1
  __SEL__Tire.ContactPointPos_wrt_WheelCenter(WorldSys)[m] : Selector  InputPortWidth=1  IndexOptions=Index vector (dialog)  Indices=ones(3, 1)  OutputSizes=1
  __SEL__Tire.LatUnitVector(WorldSys)[-] : Selector  InputPortWidth=1  IndexOptions=Index vector (dialog)  Indices=ones(3, 1)  OutputSizes=1
  __SEL__Tire.LongUnitVector(WorldSys)[-] : Selector  InputPortWidth=1  IndexOptions=Index vector (dialog)  Indices=ones(3, 1)  OutputSizes=1
  __SEL__Tire.RoadNormalVector(WorldSys)[-] : Selector  InputPortWidth=1  IndexOptions=Index vector (dialog)  Indices=ones(3, 1)  OutputSizes=1
  __SEL__Tire.WheelCenterFrc(VehSys)[N] : Selector  InputPortWidth=1  IndexOptions=Index vector (dialog)  Indices=ones(3, 1)  OutputSizes=1
  __SEL__Tire.WheelCenterTrq(VehSys)[Nm] : Selector  InputPortWidth=1  IndexOptions=Index vector (dialog)  Indices=ones(3, 1)  OutputSizes=1
  __SRC__Tire.BoreSpd(ContactSys)[rad/s] : Constant  Value=0.0  OutDataTypeStr=Inherit: Inherit via back propagation
  __SRC__Tire.CamberAng(ContactSys)[rad] : Constant  Value=0.0  OutDataTypeStr=Inherit: Inherit via back propagation
  __SRC__Tire.CircumferentialTrq_wrt_WheelRotAxis[Nm] : Constant  Value=0.0  OutDataTypeStr=Inherit: Inherit via back propagation
  __SRC__Tire.ContactPointFrc(ContactSys)[N] : Constant  Value=0.0  OutDataTypeStr=Inherit: Inherit via back propagation
  __SRC__Tire.ContactPointPos(WorldSys)[m] : Constant  Value=0.0  OutDataTypeStr=Inherit: Inherit via back propagation
  __SRC__Tire.ContactPointPos_wrt_WheelCenter(WorldSys)[m] : Constant  Value=0.0  OutDataTypeStr=Inherit: Inherit via back propagation
  __SRC__Tire.CorneringStiff[N] : Constant  Value=0.0  OutDataTypeStr=Inherit: Inherit via back propagation
  __SRC__Tire.DynamicRadius[m] : Constant  Value=0.0  OutDataTypeStr=Inherit: Inherit via back propagation
  __SRC__Tire.LatDefl(ContactSys)[m] : Constant  Value=0.0  OutDataTypeStr=Inherit: Inherit via back propagation
  __SRC__Tire.LatSpd(ContactSys)[m/s] : Constant  Value=0.0  OutDataTypeStr=Inherit: Inherit via back propagation
  __SRC__Tire.LatUnitVector(WorldSys)[-] : Constant  Value=0.0  OutDataTypeStr=Inherit: Inherit via back propagation
  __SRC__Tire.LongFrcLeverArm_wrt_WheelRotAxis[m] : Constant  Value=0.0  OutDataTypeStr=Inherit: Inherit via back propagation
  __SRC__Tire.LongSpd(ContactSys)[m/s] : Constant  Value=0.0  OutDataTypeStr=Inherit: Inherit via back propagation
  __SRC__Tire.LongUnitVector(WorldSys)[-] : Constant  Value=0.0  OutDataTypeStr=Inherit: Inherit via back propagation
  __SRC__Tire.MaxRollResistTrq[Nm] : Constant  Value=0.0  OutDataTypeStr=Inherit: Inherit via back propagation
  __SRC__Tire.RimRadius[m] : Constant  Value=0.0  OutDataTypeStr=Inherit: Inherit via back propagation
  __SRC__Tire.RoadFrictionScalingCoeff[-] : Constant  Value=0.0  OutDataTypeStr=Inherit: Inherit via back propagation
  __SRC__Tire.RoadIncl(WorldSys)[-] : Constant  Value=0.0  OutDataTypeStr=Inherit: Inherit via back propagation
  __SRC__Tire.RoadNormalVector(WorldSys)[-] : Constant  Value=0.0  OutDataTypeStr=Inherit: Inherit via back propagation
  __SRC__Tire.RoadSlope(WorldSys)[-] : Constant  Value=0.0  OutDataTypeStr=Inherit: Inherit via back propagation
  __SRC__Tire.RoadType[-] : Constant  Value=0.0  OutDataTypeStr=Inherit: Inherit via back propagation
  __SRC__Tire.Stabilization.DerivativeOfBoreTrq_wrt_BoreSpd(ContactSys)[Nm/(rad/s)] : Constant  Value=0.0  OutDataTypeStr=Inherit: Inherit via back propagation
  __SRC__Tire.Stabilization.DerivativeOfLatFrc_wrt_LatSpd(ContactSys)[N/(m/s)] : Constant  Value=0.0  OutDataTypeStr=Inherit: Inherit via back propagation
  __SRC__Tire.Stabilization.DerivativeOfLatTrq_wrt_LatSpd(ContactSys)[Nm/(m/s)] : Constant  Value=0.0  OutDataTypeStr=Inherit: Inherit via back propagation
  __SRC__Tire.Stabilization.DerivativeOfLongFrc_wrt_LongSpd(ContactSys)[N/(m/s)] : Constant  Value=0.0  OutDataTypeStr=Inherit: Inherit via back propagation
  __SRC__Tire.Stabilization.DerivativeOfLongTrq_wrt_LongSpd(ContactSys)[Nm/(m/s)] : Constant  Value=0.0  OutDataTypeStr=Inherit: Inherit via back propagation
  __SRC__Tire.TireDeflSpd[m/s] : Constant  Value=0.0  OutDataTypeStr=Inherit: Inherit via back propagation
  __SRC__Tire.TireDefl[m] : Constant  Value=0.0  OutDataTypeStr=Inherit: Inherit via back propagation
  __SRC__Tire.UnloadedRadius[m] : Constant  Value=0.0  OutDataTypeStr=Inherit: Inherit via back propagation
  __SRC__Tire.VertStiff[N/m] : Constant  Value=0.0  OutDataTypeStr=Inherit: Inherit via back propagation
  __SRC__Tire.WheelCenterFrc(VehSys)[N] : Constant  Value=0.0  OutDataTypeStr=Inherit: Inherit via back propagation
  __SRC__Tire.WheelCenterTrq(VehSys)[Nm] : Constant  Value=0.0  OutDataTypeStr=Inherit: Inherit via back propagation
  __SRC__Tire.Width[m] : Constant  Value=0.0  OutDataTypeStr=Inherit: Inherit via back propagation
  __TDO__Tire : BusCreator  Inputs=29
  __TDO__Tire.Stabilization : BusCreator  Inputs=5
  Tire___UNIQUE_1 : Outport  Description=|  PortDimensions=[49]  VectorParamsAs1DForOutWhenUnconnected=off
      | <name></name>
      | <comment></comment>
  wires:
  __SRC__Tire.ContactPointPos_wrt_WheelCenter(WorldSys)[m]/1 -> __SEL__Tire.ContactPointPos_wrt_WheelCenter(WorldSys)[m]/1
  __SRC__Tire.LongUnitVector(WorldSys)[-]/1 -> __SEL__Tire.LongUnitVector(WorldSys)[-]/1
  __SRC__Tire.LatUnitVector(WorldSys)[-]/1 -> __SEL__Tire.LatUnitVector(WorldSys)[-]/1
  __SRC__Tire.RoadNormalVector(WorldSys)[-]/1 -> __SEL__Tire.RoadNormalVector(WorldSys)[-]/1
  __SRC__Tire.ContactPointPos(WorldSys)[m]/1 -> __SEL__Tire.ContactPointPos(WorldSys)[m]/1
  __SRC__Tire.WheelCenterFrc(VehSys)[N]/1 -> __SEL__Tire.WheelCenterFrc(VehSys)[N]/1
  __SRC__Tire.WheelCenterTrq(VehSys)[Nm]/1 -> __SEL__Tire.WheelCenterTrq(VehSys)[Nm]/1
  __SRC__Tire.ContactPointFrc(ContactSys)[N]/1 -> __SEL__Tire.ContactPointFrc(ContactSys)[N]/1
  __SEL__Tire.ContactPointPos_wrt_WheelCenter(WorldSys)[m]/1 -> __TDO__Tire/1  "ContactPointPos_wrt_WheelCenter(WorldSys)[m]"
  __SRC__Tire.CamberAng(ContactSys)[rad]/1 -> __TDO__Tire/2  "CamberAng(ContactSys)[rad]"
  __SRC__Tire.TireDefl[m]/1 -> __TDO__Tire/3  "TireDefl[m]"
  __SRC__Tire.TireDeflSpd[m/s]/1 -> __TDO__Tire/4  "TireDeflSpd[m/s]"
  __SRC__Tire.LongSpd(ContactSys)[m/s]/1 -> __TDO__Tire/5  "LongSpd(ContactSys)[m/s]"
  __SRC__Tire.LatSpd(ContactSys)[m/s]/1 -> __TDO__Tire/6  "LatSpd(ContactSys)[m/s]"
  __SRC__Tire.BoreSpd(ContactSys)[rad/s]/1 -> __TDO__Tire/7  "BoreSpd(ContactSys)[rad/s]"
  __SRC__Tire.LongFrcLeverArm_wrt_WheelRotAxis[m]/1 -> __TDO__Tire/8  "LongFrcLeverArm_wrt_WheelRotAxis[m]"
  __SEL__Tire.LongUnitVector(WorldSys)[-]/1 -> __TDO__Tire/9  "LongUnitVector(WorldSys)[-]"
  __SEL__Tire.LatUnitVector(WorldSys)[-]/1 -> __TDO__Tire/10  "LatUnitVector(WorldSys)[-]"
  __SEL__Tire.RoadNormalVector(WorldSys)[-]/1 -> __TDO__Tire/11  "RoadNormalVector(WorldSys)[-]"
  __SRC__Tire.RoadType[-]/1 -> __TDO__Tire/12  "RoadType[-]"
  __SRC__Tire.RoadFrictionScalingCoeff[-]/1 -> __TDO__Tire/13  "RoadFrictionScalingCoeff[-]"
  __SEL__Tire.ContactPointPos(WorldSys)[m]/1 -> __TDO__Tire/14  "ContactPointPos(WorldSys)[m]"
  __SRC__Tire.RoadSlope(WorldSys)[-]/1 -> __TDO__Tire/15  "RoadSlope(WorldSys)[-]"
  __SRC__Tire.RoadIncl(WorldSys)[-]/1 -> __TDO__Tire/16  "RoadIncl(WorldSys)[-]"
  __SEL__Tire.WheelCenterFrc(VehSys)[N]/1 -> __TDO__Tire/17  "WheelCenterFrc(VehSys)[N]"
  __SEL__Tire.WheelCenterTrq(VehSys)[Nm]/1 -> __TDO__Tire/18  "WheelCenterTrq(VehSys)[Nm]"
  __SRC__Tire.Stabilization.DerivativeOfLongFrc_wrt_LongSpd(ContactSys)[N/(m/s)]/1 -> __TDO__Tire.Stabilization/1  "DerivativeOfLongFrc_wrt_LongSpd(ContactSys)[N/(m/s)]"
  __TDO__Tire.Stabilization/1 -> __TDO__Tire/19  "Stabilization"
  __SRC__Tire.Stabilization.DerivativeOfLongTrq_wrt_LongSpd(ContactSys)[Nm/(m/s)]/1 -> __TDO__Tire.Stabilization/2  "DerivativeOfLongTrq_wrt_LongSpd(ContactSys)[Nm/(m/s)]"
  __SRC__Tire.Stabilization.DerivativeOfLatFrc_wrt_LatSpd(ContactSys)[N/(m/s)]/1 -> __TDO__Tire.Stabilization/3  "DerivativeOfLatFrc_wrt_LatSpd(ContactSys)[N/(m/s)]"
  __SRC__Tire.Stabilization.DerivativeOfLatTrq_wrt_LatSpd(ContactSys)[Nm/(m/s)]/1 -> __TDO__Tire.Stabilization/4  "DerivativeOfLatTrq_wrt_LatSpd(ContactSys)[Nm/(m/s)]"
  __SRC__Tire.Stabilization.DerivativeOfBoreTrq_wrt_BoreSpd(ContactSys)[Nm/(rad/s)]/1 -> __TDO__Tire.Stabilization/5  "DerivativeOfBoreTrq_wrt_BoreSpd(ContactSys)[Nm/(rad/s)]"
  __SRC__Tire.CircumferentialTrq_wrt_WheelRotAxis[Nm]/1 -> __TDO__Tire/20  "CircumferentialTrq_wrt_WheelRotAxis[Nm]"
  __SRC__Tire.MaxRollResistTrq[Nm]/1 -> __TDO__Tire/21  "MaxRollResistTrq[Nm]"
  __SRC__Tire.LatDefl(ContactSys)[m]/1 -> __TDO__Tire/22  "LatDefl(ContactSys)[m]"
  __SRC__Tire.VertStiff[N/m]/1 -> __TDO__Tire/23  "VertStiff[N/m]"
  __SRC__Tire.UnloadedRadius[m]/1 -> __TDO__Tire/24  "UnloadedRadius[m]"
  __SRC__Tire.RimRadius[m]/1 -> __TDO__Tire/25  "RimRadius[m]"
  __SRC__Tire.Width[m]/1 -> __TDO__Tire/26  "Width[m]"
  __SEL__Tire.ContactPointFrc(ContactSys)[N]/1 -> __TDO__Tire/27  "ContactPointFrc(ContactSys)[N]"
  __SRC__Tire.CorneringStiff[N]/1 -> __TDO__Tire/28  "CorneringStiff[N]"
  __SRC__Tire.DynamicRadius[m]/1 -> __TDO__Tire/29  "DynamicRadius[m]"
  __TDO__Tire/1 -> Tire___UNIQUE_1/1  "Tire"
